simulink model "Telerobotic_Control"  (R2020a)
settings: Solver=VariableStepAuto  StartTime=0.0  StopTime=10.0  RelTol=1e-3
values from neighbouring files (symbols this model uses):
  Kd_m = 0.8    [Teleop_parameters.m]    (also in base.mat = 1; base_no_attrito.mat = 1; ci_siamo.mat = 0.005; force_control.mat = 1)
  Kp_m = 0.8    [Teleop_parameters.m]    (also in base.mat = 1; base_no_attrito.mat = 1; ci_siamo.mat = 0.01; force_control.mat = 1)
  lArm_m = 0.1    [Teleop_parameters.m]    (also in base.mat; base_no_attrito.mat; ci_siamo.mat; force_control.mat)
settings Model: Creator=gbagolin  LastModifiedBy=gbagolin

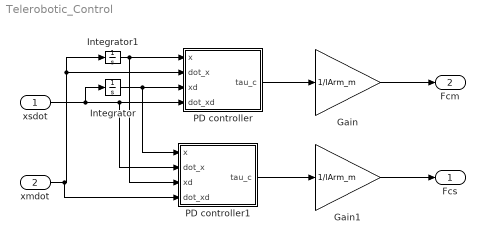
== system Telerobotic_Control ==
  xsdot : Inport
  xmdot : Inport  Port=2
  Gain : Gain  Gain=1/lArm_m
  Gain1 : Gain  Gain=1/lArm_m
  Integrator : Integrator
  Integrator1 : Integrator
  PD controller : Subsystem
  PD controller1 : Subsystem
  Fcs : Outport
  Fcm : Outport  Port=2
  wires:
  xsdot/1 -> PD controller1/2(dot_x), PD controller/4(dot_xd), Integrator/1
  Integrator/1 -> PD controller1/1(x), PD controller/3(xd)
  xmdot/1 -> PD controller1/4(dot_xd), Integrator1/1, PD controller/2(dot_x)
  Integrator1/1 -> PD controller1/3(xd), PD controller/1(x)
  PD controller/1(tau_c) -> Gain/1
  Gain/1 -> Fcm/1
  PD controller1/1(tau_c) -> Gain1/1
  Gain1/1 -> Fcs/1

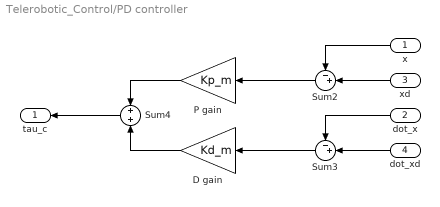
== system Telerobotic_Control/PD controller ==
  x : Inport
  dot_x : Inport  Port=2
  xd : Inport  Port=3
  dot_xd : Inport  Port=4
  D gain : Gain  Gain=Kd_m
  P gain : Gain  Gain=Kp_m
  Sum2 : Sum  Inputs=-+|
  Sum3 : Sum  Inputs=-+|
  Sum4 : Sum
  tau_c : Outport  VectorParamsAs1DForOutWhenUnconnected=off
  wires:
  D gain/1 -> Sum4/2
  dot_x/1 -> Sum3/1
  dot_xd/1 -> Sum3/2
  x/1 -> Sum2/1
  xd/1 -> Sum2/2
  Sum3/1 -> D gain/1
  P gain/1 -> Sum4/1
  Sum4/1 -> tau_c/1
  Sum2/1 -> P gain/1

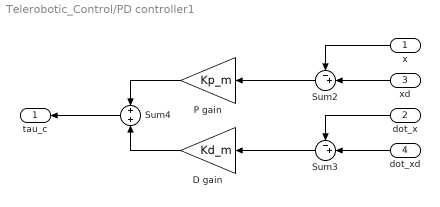
== system Telerobotic_Control/PD controller1 ==
  x : Inport
  dot_x : Inport  Port=2
  xd : Inport  Port=3
  dot_xd : Inport  Port=4
  D gain : Gain  Gain=Kd_m
  P gain : Gain  Gain=Kp_m
  Sum2 : Sum  Inputs=-+|
  Sum3 : Sum  Inputs=-+|
  Sum4 : Sum
  tau_c : Outport  VectorParamsAs1DForOutWhenUnconnected=off
  wires:
  D gain/1 -> Sum4/2
  dot_x/1 -> Sum3/1
  dot_xd/1 -> Sum3/2
  x/1 -> Sum2/1
  xd/1 -> Sum2/2
  Sum3/1 -> D gain/1
  P gain/1 -> Sum4/1
  Sum4/1 -> tau_c/1
  Sum2/1 -> P gain/1
